simulink subsystem "chute_forces"  (R2026a)
settings: Solver=VariableStepAuto
undefined symbols (not defined in the file or in its folder): chute_pos_x
settings Model: Creator=finnb  LastModifiedBy=trist

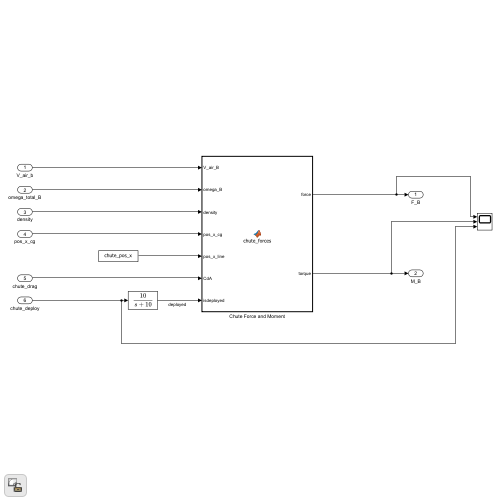
[thumbnail: Simulink's stored preview of the top-level diagram]
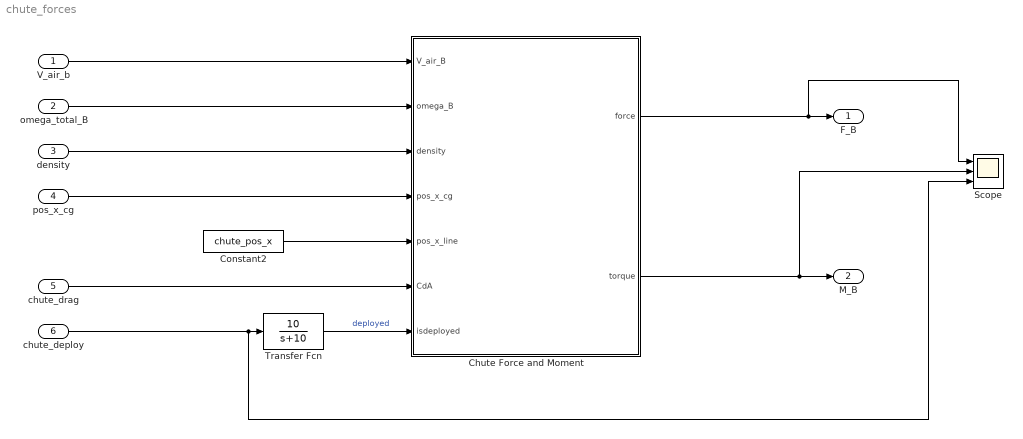
== system chute_forces ==
  V_air_b : Inport
  omega_total_B : Inport  Port=2
  "density " : Inport  Port=3
  pos_x_cg : Inport  Port=4
  chute_drag : Inport  Port=5
  chute_deploy : Inport  Port=6
  Chute Force and Moment : MATLAB Function  TreatAsAtomicUnit=on
  Constant2 : Constant  Value=chute_pos_x
  Scope : Scope  NumInputPorts=3
      settings: ActiveDisplayYMinimum=-832.42698960532493  ActiveDisplayYMaximum=1200.7071364026738  DataLoggingVariableName=ScopeData9
  Transfer Fcn : TransferFcn  Numerator=[10]  Denominator=[1 10]
  F_B : Outport
  M_B : Outport  Port=2  VectorParamsAs1DForOutWhenUnconnected=off
  wires:
  pos_x_cg/1 -> Chute Force and Moment/4(pos_x_cg)
  Constant2/1 -> Chute Force and Moment/5(pos_x_line)
  V_air_b/1 -> Chute Force and Moment/1(V_air_B)
  omega_total_B/1 -> Chute Force and Moment/2(omega_B)
  Chute Force and Moment/1(force) -> F_B/1, Scope/1
  chute_drag/1 -> Chute Force and Moment/6(CdA)
  "density "/1 -> Chute Force and Moment/3(density)
  chute_deploy/1 -> Transfer Fcn/1, Scope/3
  Transfer Fcn/1 -> Chute Force and Moment/7(isdeployed)  "deployed"
  Chute Force and Moment/2(torque) -> M_B/1, Scope/2

== matlab function chute_forces/Chute Force and Moment ==
  data: force output; V_air_B input; omega_B input; density input; pos_x_cg input; pos_x_line input; CdA input; torque output; isdeployed input
function [force, torque] = chute_forces(V_air_B, omega_B, density, pos_x_cg, pos_x_line, CdA, isdeployed)
  
    % moment arm
    pos_x = (pos_x_line - pos_x_cg) * [1;0;0];

    % relative velocity
    % V_line_B = V_air_B;
    V_line_B = V_air_B + cross(omega_B, pos_x);

    %%% Forces  
    % Chute drag force
    force_drag = - 0.5 * density * norm(V_line_B) * V_line_B * CdA;

    % damping 
    c_chute = 5; % [N*s/m], linear damping constant of chute-line system
    force_damp = -c_chute * V_line_B;

    % Total force
    force = (force_drag + force_damp) * isdeployed;
    torque = cross(pos_x, force);

end
